simulink model "f1_vehicle_model"  (R2026a)
settings: Solver=VariableStepAuto  StopTime=t_end
values from neighbouring files (symbols this model uses):
  sim_speed_real = timeseries(double(vitesse), time_seconds)    [analyse_telemetrie_f1.m]
settings Model: Creator=user  LastModifiedBy=user

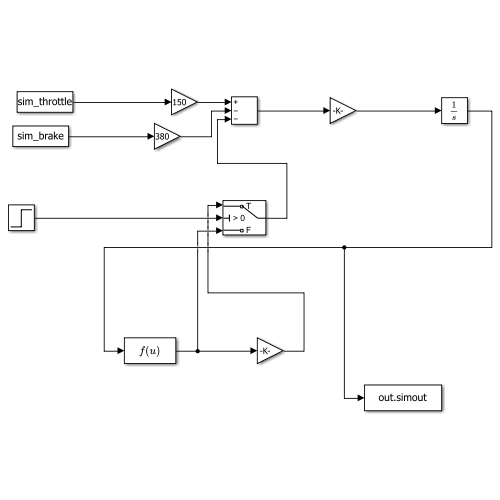
[thumbnail: Simulink's stored preview of the top-level diagram]
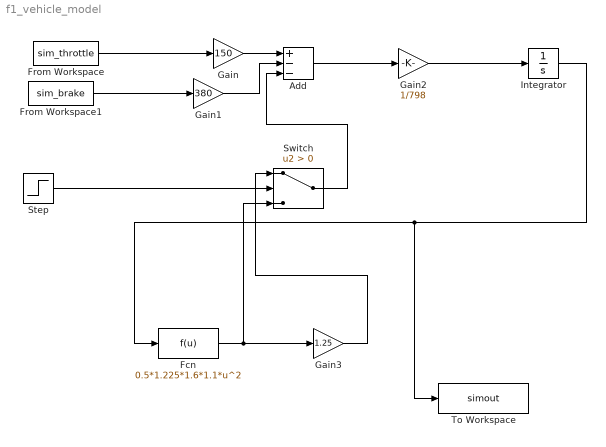
== system f1_vehicle_model ==
  Add : Sum  Inputs=+--
  Fcn : Fcn  Expr=0.5*1.225*1.6*1.1*u^2
  From Workspace : FromWorkspace  VariableName=sim_throttle
  From Workspace1 : FromWorkspace  VariableName=sim_brake
  Gain : Gain  Gain=150
  Gain1 : Gain  Gain=380
  Gain2 : Gain  Gain=1/798
  Gain3 : Gain  Gain=1.25
  Integrator : Integrator  InitialCondition=sim_speed_real.Data(1)/3.6
  Step : Step  SampleTime=0
  Switch : Switch  Criteria=u2 > Threshold  SaturateOnIntegerOverflow=off  InputSameDT=off
  To Workspace : ToWorkspace  VariableName=simout  SaveFormat=Timeseries  SampleTime=-1
  wires:
  From Workspace/1 -> Gain/1
  From Workspace1/1 -> Gain1/1
  Step/1 -> Switch/2
  Gain/1 -> Add/1
  Gain1/1 -> Add/2
  Switch/1 -> Add/3
  Add/1 -> Gain2/1
  Gain2/1 -> Integrator/1
  Integrator/1 -> Fcn/1, To Workspace/1
  Fcn/1 -> Switch/3, Gain3/1
  Gain3/1 -> Switch/1
